simulink model "DrvDem_SelectParameter"  (R2016b)
settings: configuration reference "CodeGenConfigSet" (kept outside this file)
values from neighbouring files (symbols this model uses):
  DrvDem_dnAccLim_CUR = Calibration.Parameter    [init_DrvDem_SelectParameter.m]
  DrvDem_dnAccLim_CURX = Calibration.Parameter    [init_DrvDem_SelectParameter.m]
  DrvDem_dnDeclLim_CUR = Calibration.Parameter    [init_DrvDem_SelectParameter.m]
  DrvDem_dnDeclLim_CURX = Calibration.Parameter    [init_DrvDem_SelectParameter.m]
  DrvDem_facFdbkTrqLosHiParSet_CUR = Calibration.Parameter    [init_DrvDem_SelectParameter.m]
  DrvDem_facFdbkTrqLosHiParSet_CURX = Calibration.Parameter    [init_DrvDem_SelectParameter.m]
  DrvDem_facFdbkTrqLosLoParSet_CUR = Calibration.Parameter    [init_DrvDem_SelectParameter.m]
  DrvDem_facFdbkTrqLosLoParSet_CURX = Calibration.Parameter    [init_DrvDem_SelectParameter.m]
  DrvDem_facNAvrgPT1CorFac_C = Calibration.Parameter    [init_DrvDem_SelectParameter.m]
  DrvDem_facTrqPT1CorFac_C = Calibration.Parameter    [init_DrvDem_SelectParameter.m]
  DrvDem_KiCorTempFac_MAP = Calibration.Parameter    [init_DrvDem_SelectParameter.m]
  DrvDem_KiCorTempFac_MAPX = Calibration.Parameter    [init_DrvDem_SelectParameter.m]
  DrvDem_KiCorTempFac_MAPY = Calibration.Parameter    [init_DrvDem_SelectParameter.m]
  DrvDem_KiCorTrqFac_MAP = Calibration.Parameter    [init_DrvDem_SelectParameter.m]
  DrvDem_KiCorTrqFac_MAPX = Calibration.Parameter    [init_DrvDem_SelectParameter.m]
  DrvDem_KiCorTrqFac_MAPY = Calibration.Parameter    [init_DrvDem_SelectParameter.m]
  DrvDem_KpCorTempFac_MAP = Calibration.Parameter    [init_DrvDem_SelectParameter.m]
  DrvDem_KpCorTempFac_MAPX = Calibration.Parameter    [init_DrvDem_SelectParameter.m]
  DrvDem_KpCorTempFac_MAPY = Calibration.Parameter    [init_DrvDem_SelectParameter.m]
  DrvDem_KpCorTrqFac_MAP = Calibration.Parameter    [init_DrvDem_SelectParameter.m]
  DrvDem_KpCorTrqFac_MAPX = Calibration.Parameter    [init_DrvDem_SelectParameter.m]
  DrvDem_KpCorTrqFac_MAPY = Calibration.Parameter    [init_DrvDem_SelectParameter.m]
  DrvDem_ParSetIKiLo_CUR = Calibration.Parameter    [init_DrvDem_SelectParameter.m]
  DrvDem_ParSetIKiLo_CURX = Calibration.Parameter    [init_DrvDem_SelectParameter.m]
  DrvDem_ParSetIKiNegLo_CUR = Calibration.Parameter    [init_DrvDem_SelectParameter.m]
  DrvDem_ParSetIKiNegLo_CURX = Calibration.Parameter    [init_DrvDem_SelectParameter.m]
  DrvDem_ParSetIKiPosLo_CUR = Calibration.Parameter    [init_DrvDem_SelectParameter.m]
  DrvDem_ParSetIKiPosLo_CURX = Calibration.Parameter    [init_DrvDem_SelectParameter.m]
  DrvDem_ParSetInrtVeh_CUR = Calibration.Parameter    [init_DrvDem_SelectParameter.m]
  DrvDem_ParSetInrtVeh_CURX = Calibration.Parameter    [init_DrvDem_SelectParameter.m]
  DrvDem_ParSetIWinNegHi_C = Calibration.Parameter    [init_DrvDem_SelectParameter.m]
  DrvDem_ParSetIWinNegLo_C = Calibration.Parameter    [init_DrvDem_SelectParameter.m]
  DrvDem_ParSetIWinPosHi_C = Calibration.Parameter    [init_DrvDem_SelectParameter.m]
  DrvDem_ParSetIWinPosLo_C = Calibration.Parameter    [init_DrvDem_SelectParameter.m]
  DrvDem_ParSetPKpLo_CUR = Calibration.Parameter    [init_DrvDem_SelectParameter.m]
  DrvDem_ParSetPKpLo_CURX = Calibration.Parameter    [init_DrvDem_SelectParameter.m]
  DrvDem_ParSetPKpNegLo_CUR = Calibration.Parameter    [init_DrvDem_SelectParameter.m]
  DrvDem_ParSetPKpNegLo_CURX = Calibration.Parameter    [init_DrvDem_SelectParameter.m]
  DrvDem_ParSetPKpPosLo_CUR = Calibration.Parameter    [init_DrvDem_SelectParameter.m]
  DrvDem_ParSetPKpPosLo_CURX = Calibration.Parameter    [init_DrvDem_SelectParameter.m]
  DrvDem_ParSetPWinNegHi_C = Calibration.Parameter    [init_DrvDem_SelectParameter.m]
  DrvDem_ParSetPWinNegLo_C = Calibration.Parameter    [init_DrvDem_SelectParameter.m]
  DrvDem_ParSetPWinPosHi_C = Calibration.Parameter    [init_DrvDem_SelectParameter.m]
  DrvDem_ParSetPWinPosLo_C = Calibration.Parameter    [init_DrvDem_SelectParameter.m]
  DrvDem_ParSetTiFltTrqLos_CUR = Calibration.Parameter    [init_DrvDem_SelectParameter.m]
  DrvDem_ParSetTiFltTrqLos_CURX = Calibration.Parameter    [init_DrvDem_SelectParameter.m]
  DrvDem_swtTempSelParAdap_C = Calibration.Parameter    [init_DrvDem_SelectParameter.m]
  DrvDem_swtTrqSelCorFac_C = Calibration.Parameter    [init_DrvDem_SelectParameter.m]
undefined symbols (not defined in the file or in its folder): DrvDem_SelectParameter_DT, HLSDem_KpCorFac_MAPX
libraries: CXLib x4
settings Model: Creator=lenovo  LastModifiedBy=xuxingpei
settings ConfigSetRef: SourceLocation=Base Workspace

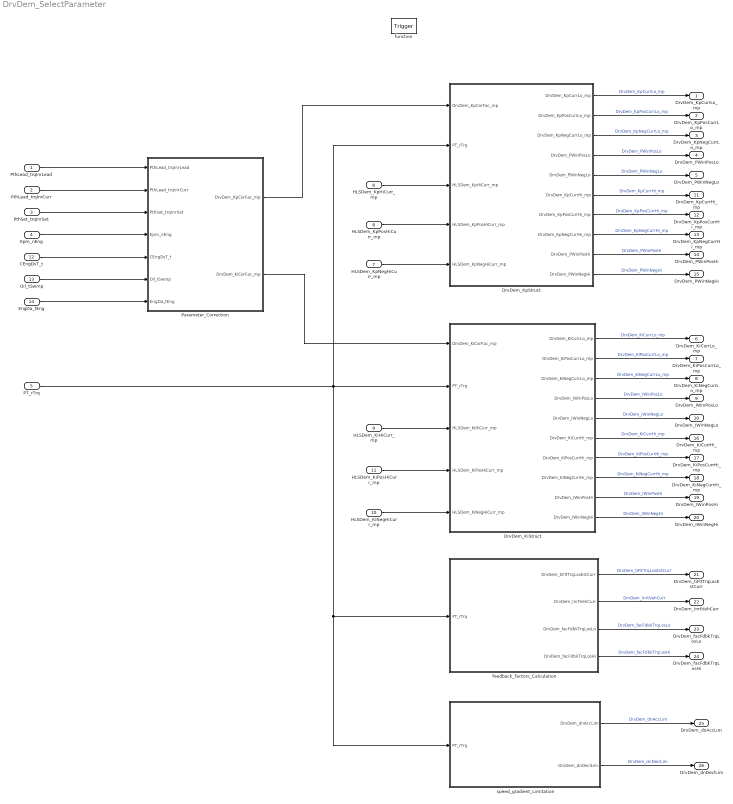
== system DrvDem_SelectParameter ==
  PthLead_trqInrLead : Inport  Tag=Nm  Description=Inner torque lead value  OutMin=-3000  OutMax=3000  OutDataTypeStr=Trq_Nm
  PthLead_trqInrCurr : Inport  Tag=Nm  Description=Actual percent engine torque  Port=2  OutMin=-3000  OutMax=3000  OutDataTypeStr=Trq_Nm
  PthSet_trqInrSet : Inport  Tag=Nm  Description=Inner torque set value after monitoring limitation  Port=3  OutMin=-3000  OutMax=3276.7  OutDataTypeStr=Trq_Nm
  Epm_nEng : Inport  Tag=rpm  Description=Engine speed  Port=4  OutMin=0  OutMax=6000  OutDataTypeStr=EngSpeed_rpm
  PT_rTrq : Inport  Description=Powertrain torque ratio  Port=5  OutMin=-100  OutMax=100  OutDataTypeStr=TransRatio
  HLSDem_KpHiCurr_mp : Inport  Tag=Nm/rpm  Description=Current gain of the P-element of upper path  Port=6  OutMin=-10000  OutMax=10000  OutDataTypeStr=HLSDem_Kp
  HLSDem_KpNegHiCurr_mp : Inport  Tag=Nm/rpm  Description=Current negative large signal gain of the P-element of upper path  Port=7  OutMin=-10000  OutMax=10000  OutDataTypeStr=HLSDem_Kp
  HLSDem_KpPosHiCurr_mp : Inport  Tag=Nm/rpm  Description=Current positive large signal gain of the P-element of upper path  Port=8  OutMin=-10000  OutMax=10000  OutDataTypeStr=HLSDem_Kp
  HLSDem_KiHiCurr_mp : Inport  Tag=Nm/(rpm*s)  Description=Current small signal gain for the I component upper PI - path  Port=9  OutMin=-18000  OutMax=18000  OutDataTypeStr=HLSDem_Ki
  HLSDem_KiNegHiCurr_mp : Inport  Tag=Nm/(rpm*s)  Description=Current negative large signal gain for the I component upper PI - path  Port=10  OutMin=-18000  OutMax=18000  OutDataTypeStr=HLSDem_Ki
  HLSDem_KiPosHiCurr_mp : Inport  Tag=Nm/(rpm*s)  Description=Current positive large signal gain for the I component upper PI-path  Port=11  OutMin=-18000  OutMax=18000  OutDataTypeStr=HLSDem_Ki
  CEngDsT_t : Inport  Tag=deg  Description=engine coolant temperature after filter  Port=12  OutMin=-200  OutMax=200  OutDataTypeStr=Temp_deg
  Oil_tSwmp : Inport  Tag=deg  Description=Oil temperature in oil sump  Port=13  OutMin=-50  OutMax=200  OutDataTypeStr=Temp_deg
  EngDa_tEng : Inport  Tag=deg  Description=Engine temperature  Port=14  OutMin=-1000  OutMax=1000  OutDataTypeStr=Temp_deg
  function : TriggerPort  TriggerType=function-call  VariantControl=Variant
  DrvDem_KiStruct : Subsystem
  DrvDem_KpStruct : Subsystem
  Parameter_Correction : Subsystem
  feedback_factors_Calculation : Subsystem
  speed_gradient_Limitation : Subsystem
  DrvDem_KpCurrLo_mp : Outport  Tag=Nm/rpm  Description=Current gain for the P element for the lower path  OutMin=-10000  OutMax=10000  OutDataTypeStr=HLSDem_Kp
  DrvDem_KpPosCurrLo_mp : Outport  Tag=Nm/rpm  Description=Current positive large signal gain for the P component lower PI-path  Port=2  OutMin=-10000  OutMax=10000  OutDataTypeStr=HLSDem_Kp
  DrvDem_KpNegCurrLo_mp : Outport  Tag=Nm/rpm  Description=Current negative large signal gain for the P component lower PI-path  Port=3  OutMin=-10000  OutMax=10000  OutDataTypeStr=HLSDem_Kp
  DrvDem_PWinPosLo : Outport  Tag=rpm  Description=P component Positive window for parameterset lower PI- path  Port=4  OutMin=-6000  OutMax=6000  OutDataTypeStr=EngSpeed_rpm
  DrvDem_PWinNegLo : Outport  Tag=rpm  Description=P component negative window for parameterset lower PI- path  Port=5  OutMin=-6000  OutMax=6000  OutDataTypeStr=EngSpeed_rpm
  DrvDem_KiCurrLo_mp : Outport  Tag=Nm/(rpm*s)  Description=Current gain for the I element for the lower path  Port=6  OutMin=-18000  OutMax=18000  OutDataTypeStr=HLSDem_Ki
  DrvDem_KiPosCurrLo_mp : Outport  Tag=Nm/(rpm*s)  Description=Current positive large signal gain for the I component lower PI-path  Port=7  OutMin=-18000  OutMax=18000  OutDataTypeStr=HLSDem_Ki
  DrvDem_KiNegCurrLo_mp : Outport  Tag=Nm/(rpm*s)  Description=Current negative large signal gain for the I component lower PI-path  Port=8  OutMin=-18000  OutMax=18000  OutDataTypeStr=HLSDem_Ki
  DrvDem_IWinPosLo : Outport  Tag=rpm  Description=I component Positive window for parameterset lower PI- path  Port=9  OutMin=-6000  OutMax=6000  OutDataTypeStr=EngSpeed_rpm
  DrvDem_IWinNegLo : Outport  Tag=rpm  Description=I component negative window for parameterset lower PI- path  Port=10  OutMin=-6000  OutMax=6000  OutDataTypeStr=EngSpeed_rpm
  DrvDem_KpCurrHi_mp : Outport  Tag=Nm/rpm  Description=Current gain for the P element for the upper path  Port=11  OutMin=-10000  OutMax=10000  OutDataTypeStr=HLSDem_Kp
  DrvDem_KpPosCurrHi_mp : Outport  Tag=Nm/rpm  Description=Current positive large signal gain for the P component upper PI-path  Port=12  OutMin=-10000  OutMax=10000  OutDataTypeStr=HLSDem_Kp
  DrvDem_KpNegCurrHi_mp : Outport  Tag=Nm/rpm  Description=Current negative large signal gain for the P component upper PI-path  Port=13  OutMin=-10000  OutMax=10000  OutDataTypeStr=HLSDem_Kp
  DrvDem_PWinPosHi : Outport  Tag=rpm  Description=P component Positive window for parameterset upper PI- path  Port=14  OutMin=-6000  OutMax=6000  OutDataTypeStr=EngSpeed_rpm
  DrvDem_PWinNegHi : Outport  Tag=rpm  Description=P component negative window for parameterset upper PI- path  Port=15  OutMin=-6000  OutMax=6000  OutDataTypeStr=EngSpeed_rpm
  DrvDem_KiCurrHi_mp : Outport  Tag=Nm/(rpm*s)  Description=Current gain for the I element for the upper path  Port=16  OutMin=-18000  OutMax=18000  OutDataTypeStr=HLSDem_Ki
  DrvDem_KiPosCurrHi_mp : Outport  Tag=Nm/(rpm*s)  Description=Current positive large signal gain for the I component upper PI-path  Port=17  OutMin=-18000  OutMax=18000  OutDataTypeStr=HLSDem_Ki
  DrvDem_KiNegCurrHi_mp : Outport  Tag=Nm/(rpm*s)  Description=Current negative large signal gain for the I component upper PI-path  Port=18  OutMin=-18000  OutMax=18000  OutDataTypeStr=HLSDem_Ki
  DrvDem_IWinPosHi : Outport  Tag=rpm  Description=I component Positive window for parameterset upper PI- path  Port=19  OutMin=-6000  OutMax=6000  OutDataTypeStr=EngSpeed_rpm
  DrvDem_IWinNegHi : Outport  Tag=rpm  Description=I component negative window for parameterset upper PI- path  Port=20  OutMin=-6000  OutMax=6000  OutDataTypeStr=EngSpeed_rpm
  DrvDem_tiFltTrqLosEstCurr : Outport  Description=Time constant (PT1filter) for EISGov torque loss estimation  Port=21  OutMin=0  OutMax=99.998  OutDataTypeStr=PT_fac
  DrvDem_InrtVehCurr : Outport  Tag=Nm/(rpm/s)  Description=Mass Inertia for EISGov torque loss estimation  Port=22  OutMin=-50  OutMax=50  OutDataTypeStr=HLSDem_Inrt
  DrvDem_facFdbkTrqLosLo : Outport  Tag=rpm/Nm  Description=Inner feedback factor for the lower setpoint  Port=23  OutMin=-20  OutMax=20  OutDataTypeStr=FdbkNm2rpm_rpm_Nm
  DrvDem_facFdbkTrqLosHi : Outport  Tag=rpm/Nm  Description=Inner feedback factor for the upper setpoint  Port=24  OutMin=-20  OutMax=20  OutDataTypeStr=FdbkNm2rpm_rpm_Nm
  DrvDem_dnAccLim : Outport  Tag=rpm/s  Description=Maximum permissible acceleration (Engine speed)  Port=25  OutMin=-12000  OutMax=12000  OutDataTypeStr=EngSpeed_rpm_s
  DrvDem_dnDeclLim : Outport  Tag=rpm/s  Description=Maximum permissible deceleration (Engine speed)  Port=26  OutMin=-12000  OutMax=12000  OutDataTypeStr=EngSpeed_rpm_s
  wires:
  PthLead_trqInrLead/1 -> Parameter_Correction/1(PthLead_trqInrLead)
  PthLead_trqInrCurr/1 -> Parameter_Correction/2(PthLead_trqInrCurr)
  PthSet_trqInrSet/1 -> Parameter_Correction/3(PthSet_trqInrSet)
  Epm_nEng/1 -> Parameter_Correction/4(Epm_nEng)
  CEngDsT_t/1 -> Parameter_Correction/5(CEngDsT_t)
  Oil_tSwmp/1 -> Parameter_Correction/6(Oil_tSwmp)
  EngDa_tEng/1 -> Parameter_Correction/7(EngDa_tEng)
  PT_rTrq/1 -> speed_gradient_Limitation/1(PT_rTrq), feedback_factors_Calculation/1(PT_rTrq), DrvDem_KpStruct/2(PT_rTrq), DrvDem_KiStruct/2(PT_rTrq)
  Parameter_Correction/1(DrvDem_KpCorFac_mp) -> DrvDem_KpStruct/1(DrvDem_KpCorFac_mp)
  HLSDem_KpHiCurr_mp/1 -> DrvDem_KpStruct/3(HLSDem_KpHiCurr_mp)
  HLSDem_KpPosHiCurr_mp/1 -> DrvDem_KpStruct/4(HLSDem_KpPosHiCurr_mp)
  HLSDem_KpNegHiCurr_mp/1 -> DrvDem_KpStruct/5(HLSDem_KpNegHiCurr_mp)
  DrvDem_KpStruct/1(DrvDem_KpCurrLo_mp) -> DrvDem_KpCurrLo_mp/1  "DrvDem_KpCurrLo_mp"
  DrvDem_KpStruct/2(DrvDem_KpPosCurrLo_mp) -> DrvDem_KpPosCurrLo_mp/1  "DrvDem_KpPosCurrLo_mp"
  DrvDem_KpStruct/3(DrvDem_KpNegCurrLo_mp) -> DrvDem_KpNegCurrLo_mp/1  "DrvDem_KpNegCurrLo_mp"
  DrvDem_KpStruct/4(DrvDem_PWinPosLo) -> DrvDem_PWinPosLo/1  "DrvDem_PWinPosLo"
  DrvDem_KpStruct/5(DrvDem_PWinNegLo) -> DrvDem_PWinNegLo/1  "DrvDem_PWinNegLo"
  DrvDem_KpStruct/6(DrvDem_KpCurrHi_mp) -> DrvDem_KpCurrHi_mp/1  "DrvDem_KpCurrHi_mp"
  DrvDem_KpStruct/7(DrvDem_KpPosCurrHi_mp) -> DrvDem_KpPosCurrHi_mp/1  "DrvDem_KpPosCurrHi_mp"
  DrvDem_KpStruct/8(DrvDem_KpNegCurrHi_mp) -> DrvDem_KpNegCurrHi_mp/1  "DrvDem_KpNegCurrHi_mp"
  DrvDem_KpStruct/9(DrvDem_PWinPosHi) -> DrvDem_PWinPosHi/1  "DrvDem_PWinPosHi"
  DrvDem_KpStruct/10(DrvDem_PWinNegHi) -> DrvDem_PWinNegHi/1  "DrvDem_PWinNegHi"
  HLSDem_KiHiCurr_mp/1 -> DrvDem_KiStruct/3(HLSDem_KiHiCurr_mp)
  DrvDem_KiStruct/1(DrvDem_KiCurrLo_mp) -> DrvDem_KiCurrLo_mp/1  "DrvDem_KiCurrLo_mp"
  DrvDem_KiStruct/2(DrvDem_KiPosCurrLo_mp) -> DrvDem_KiPosCurrLo_mp/1  "DrvDem_KiPosCurrLo_mp"
  DrvDem_KiStruct/3(DrvDem_KiNegCurrLo_mp) -> DrvDem_KiNegCurrLo_mp/1  "DrvDem_KiNegCurrLo_mp"
  DrvDem_KiStruct/4(DrvDem_IWinPosLo) -> DrvDem_IWinPosLo/1  "DrvDem_IWinPosLo"
  DrvDem_KiStruct/5(DrvDem_IWinNegLo) -> DrvDem_IWinNegLo/1  "DrvDem_IWinNegLo"
  DrvDem_KiStruct/6(DrvDem_KiCurrHi_mp) -> DrvDem_KiCurrHi_mp/1  "DrvDem_KiCurrHi_mp"
  DrvDem_KiStruct/7(DrvDem_KiPosCurrHi_mp) -> DrvDem_KiPosCurrHi_mp/1  "DrvDem_KiPosCurrHi_mp"
  DrvDem_KiStruct/8(DrvDem_KiNegCurrHi_mp) -> DrvDem_KiNegCurrHi_mp/1  "DrvDem_KiNegCurrHi_mp"
  DrvDem_KiStruct/9(DrvDem_IWinPosHi) -> DrvDem_IWinPosHi/1  "DrvDem_IWinPosHi"
  DrvDem_KiStruct/10(DrvDem_IWinNegHi) -> DrvDem_IWinNegHi/1  "DrvDem_IWinNegHi"
  feedback_factors_Calculation/1(DrvDem_tiFltTrqLosEstCurr) -> DrvDem_tiFltTrqLosEstCurr/1  "DrvDem_tiFltTrqLosEstCurr"
  feedback_factors_Calculation/2(DrvDem_InrtVehCurr) -> DrvDem_InrtVehCurr/1  "DrvDem_InrtVehCurr"
  feedback_factors_Calculation/3(DrvDem_facFdbkTrqLosLo) -> DrvDem_facFdbkTrqLosLo/1  "DrvDem_facFdbkTrqLosLo"
  feedback_factors_Calculation/4(DrvDem_facFdbkTrqLosHi) -> DrvDem_facFdbkTrqLosHi/1  "DrvDem_facFdbkTrqLosHi"
  speed_gradient_Limitation/1(DrvDem_dnAccLim) -> DrvDem_dnAccLim/1  "DrvDem_dnAccLim"
  speed_gradient_Limitation/2(DrvDem_dnDeclLim) -> DrvDem_dnDeclLim/1  "DrvDem_dnDeclLim"
  Parameter_Correction/2(DrvDem_KiCorFac_mp) -> DrvDem_KiStruct/1(DrvDem_KiCorFac_mp)
  HLSDem_KiPosHiCurr_mp/1 -> DrvDem_KiStruct/4(HLSDem_KiPosHiCurr_mp)
  HLSDem_KiNegHiCurr_mp/1 -> DrvDem_KiStruct/5(HLSDem_KiNegHiCurr_mp)

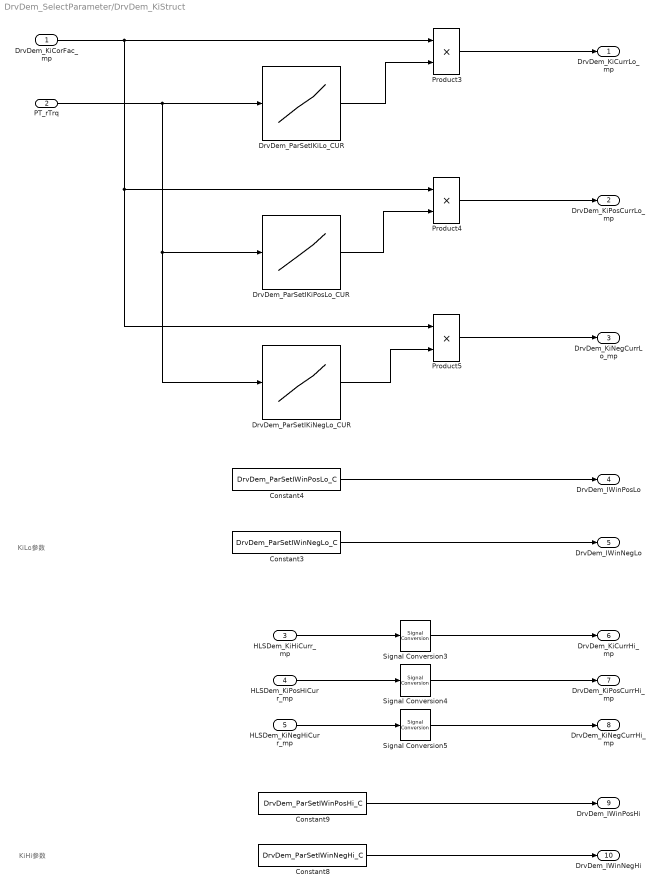
== system DrvDem_SelectParameter/DrvDem_KiStruct ==
  note: KiLo参数
  note: KiHi参数
  DrvDem_KiCorFac_mp : Inport
  PT_rTrq : Inport  Port=2
  HLSDem_KiHiCurr_mp : Inport  Tag=Nm/(rpm*s)  Description=Current small signal gain for the I component upper PI - path  Port=3
  HLSDem_KiPosHiCurr_mp : Inport  Tag=Nm/(rpm*s)  Description=Current positive large signal gain for the I component upper PI-path  Port=4
  HLSDem_KiNegHiCurr_mp : Inport  Tag=Nm/(rpm*s)  Description=Current negative large signal gain for the I component upper PI - path  Port=5
  Constant3 : Constant  Value=DrvDem_ParSetIWinNegLo_C  SampleTime=-1
  Constant4 : Constant  Value=DrvDem_ParSetIWinPosLo_C  SampleTime=-1
  Constant8 : Constant  Value=DrvDem_ParSetIWinNegHi_C  SampleTime=-1
  Constant9 : Constant  Value=DrvDem_ParSetIWinPosHi_C  SampleTime=-1
  DrvDem_ParSetIKiLo_CUR : Lookup_n-D  NumberOfTableDimensions=1  BreakpointsForDimension1=DrvDem_ParSetIKiLo_CURX  BreakpointsForDimension2=HLSDem_KpCorFac_MAPX  Table=DrvDem_ParSetIKiLo_CUR  ExtrapMethod=Clip  InternalRulePriority=Speed  OutDataTypeStr=Inherit: Inherit via back propagation  RndMeth=Simplest  SaturateOnIntegerOverflow=on
  DrvDem_ParSetIKiNegLo_CUR : Lookup_n-D  NumberOfTableDimensions=1  BreakpointsForDimension1=DrvDem_ParSetIKiNegLo_CURX  BreakpointsForDimension2=HLSDem_KpCorFac_MAPX  Table=DrvDem_ParSetIKiNegLo_CUR  ExtrapMethod=Clip  InternalRulePriority=Speed  OutDataTypeStr=Inherit: Inherit via back propagation  RndMeth=Simplest  SaturateOnIntegerOverflow=on
  DrvDem_ParSetIKiPosLo_CUR : Lookup_n-D  NumberOfTableDimensions=1  BreakpointsForDimension1=DrvDem_ParSetIKiPosLo_CURX  BreakpointsForDimension2=HLSDem_KpCorFac_MAPX  Table=DrvDem_ParSetIKiPosLo_CUR  ExtrapMethod=Clip  InternalRulePriority=Speed  OutDataTypeStr=Inherit: Inherit via back propagation  RndMeth=Simplest  SaturateOnIntegerOverflow=on
  Product3 : Product  OutDataTypeStr=Inherit: Inherit via back propagation
  Product4 : Product  OutDataTypeStr=Inherit: Inherit via back propagation
  Product5 : Product  OutDataTypeStr=Inherit: Inherit via back propagation
  Signal Conversion3 : SignalConversion  OverrideOpt=off
  Signal Conversion4 : SignalConversion  OverrideOpt=off
  Signal Conversion5 : SignalConversion  OverrideOpt=off
  DrvDem_KiCurrLo_mp : Outport  Tag=Nm/(rpm*s)  Description=Current gain for the I element for the lower path  OutMin=-18000  OutMax=18000  OutDataTypeStr=HLSDem_Ki
  DrvDem_KiPosCurrLo_mp : Outport  Tag=Nm/(rpm*s)  Description=Current positive large signal gain for the I component lower PI-path  Port=2  OutMin=-18000  OutMax=18000  OutDataTypeStr=HLSDem_Ki
  DrvDem_KiNegCurrLo_mp : Outport  Tag=Nm/(rpm*s)  Description=Current negative large signal gain for the I component lower PI-path  Port=3  OutMin=-18000  OutMax=18000  OutDataTypeStr=HLSDem_Ki
  DrvDem_IWinPosLo : Outport  Tag=rpm  Description=I component Positive window for parameterset lower PI- path  Port=4  OutMin=-6000  OutMax=6000  OutDataTypeStr=EngSpeed_rpm
  DrvDem_IWinNegLo : Outport  Tag=rpm  Description=I component negative window for parameterset lower PI- path  Port=5  OutMin=-6000  OutMax=6000  OutDataTypeStr=EngSpeed_rpm
  DrvDem_KiCurrHi_mp : Outport  Tag=Nm/(rpm*s)  Description=Current gain for the I element for the upper path  Port=6  OutMin=-18000  OutMax=18000  OutDataTypeStr=HLSDem_Ki
  DrvDem_KiPosCurrHi_mp : Outport  Tag=Nm/(rpm*s)  Description=Current positive large signal gain for the I component upper PI-path  Port=7  OutMin=-18000  OutMax=18000  OutDataTypeStr=HLSDem_Ki
  DrvDem_KiNegCurrHi_mp : Outport  Tag=Nm/(rpm*s)  Description=Current negative large signal gain for the I component upper PI-path  Port=8  OutMin=-18000  OutMax=18000  OutDataTypeStr=HLSDem_Ki
  DrvDem_IWinPosHi : Outport  Tag=rpm  Description=I component Positive window for parameterset upper PI- path  Port=9  OutMin=-6000  OutMax=6000  OutDataTypeStr=EngSpeed_rpm
  DrvDem_IWinNegHi : Outport  Tag=rpm  Description=I component negative window for parameterset upper PI- path  Port=10  OutMin=-6000  OutMax=6000  OutDataTypeStr=EngSpeed_rpm
  wires:
  PT_rTrq/1 -> DrvDem_ParSetIKiNegLo_CUR/1, DrvDem_ParSetIKiPosLo_CUR/1, DrvDem_ParSetIKiLo_CUR/1
  Product3/1 -> DrvDem_KiCurrLo_mp/1
  Product4/1 -> DrvDem_KiPosCurrLo_mp/1
  Product5/1 -> DrvDem_KiNegCurrLo_mp/1
  Constant4/1 -> DrvDem_IWinPosLo/1
  Constant3/1 -> DrvDem_IWinNegLo/1
  Signal Conversion3/1 -> DrvDem_KiCurrHi_mp/1
  Signal Conversion4/1 -> DrvDem_KiPosCurrHi_mp/1
  Signal Conversion5/1 -> DrvDem_KiNegCurrHi_mp/1
  DrvDem_ParSetIKiNegLo_CUR/1 -> Product5/2
  DrvDem_KiCorFac_mp/1 -> Product5/1, Product4/1, Product3/1
  DrvDem_ParSetIKiLo_CUR/1 -> Product3/2
  DrvDem_ParSetIKiPosLo_CUR/1 -> Product4/2
  HLSDem_KiHiCurr_mp/1 -> Signal Conversion3/1
  Constant8/1 -> DrvDem_IWinNegHi/1
  Constant9/1 -> DrvDem_IWinPosHi/1
  HLSDem_KiNegHiCurr_mp/1 -> Signal Conversion5/1
  HLSDem_KiPosHiCurr_mp/1 -> Signal Conversion4/1

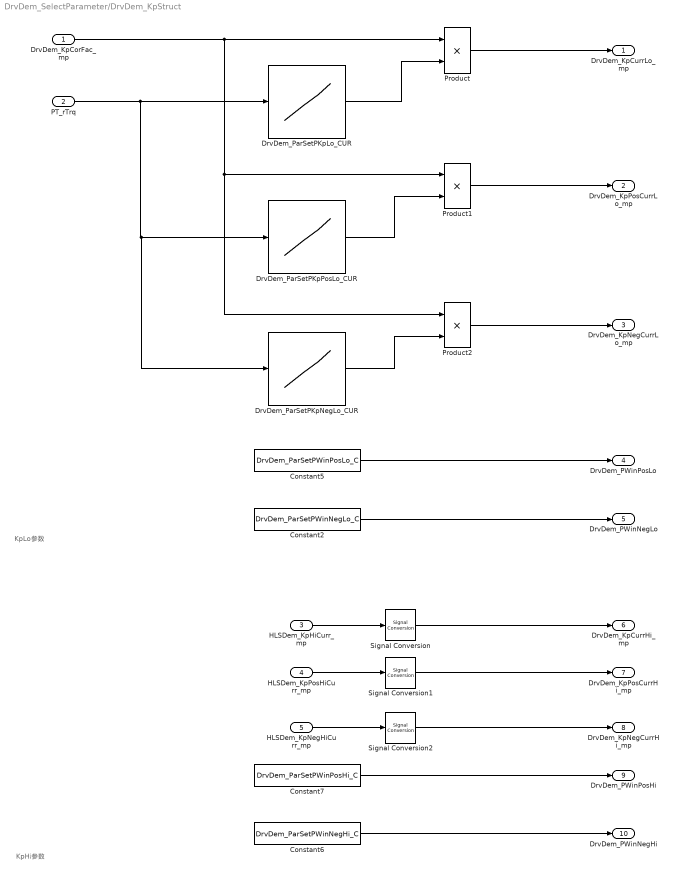
== system DrvDem_SelectParameter/DrvDem_KpStruct ==
  note: KpLo参数
  note: KpHi参数
  DrvDem_KpCorFac_mp : Inport
  PT_rTrq : Inport  Port=2
  HLSDem_KpHiCurr_mp : Inport  Tag=Nm/rpm  Description=Current gain of the P-element of upper path  Port=3
  HLSDem_KpPosHiCurr_mp : Inport  Tag=Nm/rpm  Description=Current positive large signal gain of the P-element of upper path  Port=4
  HLSDem_KpNegHiCurr_mp : Inport  Tag=Nm/rpm  Description=Current negative large signal gain of the P-element of upper path  Port=5
  Constant2 : Constant  Value=DrvDem_ParSetPWinNegLo_C  SampleTime=-1
  Constant5 : Constant  Value=DrvDem_ParSetPWinPosLo_C  SampleTime=-1
  Constant6 : Constant  Value=DrvDem_ParSetPWinNegHi_C  SampleTime=-1
  Constant7 : Constant  Value=DrvDem_ParSetPWinPosHi_C  SampleTime=-1
  DrvDem_ParSetPKpLo_CUR : Lookup_n-D  NumberOfTableDimensions=1  BreakpointsForDimension1=DrvDem_ParSetPKpLo_CURX  BreakpointsForDimension2=HLSDem_KpCorFac_MAPX  Table=DrvDem_ParSetPKpLo_CUR  ExtrapMethod=Clip  InternalRulePriority=Speed  OutDataTypeStr=Inherit: Inherit via back propagation  RndMeth=Simplest  SaturateOnIntegerOverflow=on
  DrvDem_ParSetPKpNegLo_CUR : Lookup_n-D  NumberOfTableDimensions=1  BreakpointsForDimension1=DrvDem_ParSetPKpNegLo_CURX  BreakpointsForDimension2=HLSDem_KpCorFac_MAPX  Table=DrvDem_ParSetPKpNegLo_CUR  ExtrapMethod=Clip  InternalRulePriority=Speed  OutDataTypeStr=Inherit: Inherit via back propagation  RndMeth=Simplest  SaturateOnIntegerOverflow=on
  DrvDem_ParSetPKpPosLo_CUR : Lookup_n-D  NumberOfTableDimensions=1  BreakpointsForDimension1=DrvDem_ParSetPKpPosLo_CURX  BreakpointsForDimension2=HLSDem_KpCorFac_MAPX  Table=DrvDem_ParSetPKpPosLo_CUR  ExtrapMethod=Clip  InternalRulePriority=Speed  OutDataTypeStr=Inherit: Inherit via back propagation  RndMeth=Simplest  SaturateOnIntegerOverflow=on
  Product : Product  OutDataTypeStr=Inherit: Inherit via back propagation
  Product1 : Product  OutDataTypeStr=Inherit: Inherit via back propagation
  Product2 : Product  OutDataTypeStr=Inherit: Inherit via back propagation
  Signal Conversion : SignalConversion  OverrideOpt=off
  Signal Conversion1 : SignalConversion  OverrideOpt=off
  Signal Conversion2 : SignalConversion  OverrideOpt=off
  DrvDem_KpCurrLo_mp : Outport  Tag=Nm/rpm  Description=Current gain for the P element for the lower path  OutMin=-10000  OutMax=10000  OutDataTypeStr=HLSDem_Kp
  DrvDem_KpPosCurrLo_mp : Outport  Tag=Nm/rpm  Description=Current positive large signal gain for the P component lower PI-path  Port=2  OutMin=-10000  OutMax=10000  OutDataTypeStr=HLSDem_Kp
  DrvDem_KpNegCurrLo_mp : Outport  Tag=Nm/rpm  Description=Current negative large signal gain for the P component lower PI-path  Port=3  OutMin=-10000  OutMax=10000  OutDataTypeStr=HLSDem_Kp
  DrvDem_PWinPosLo : Outport  Tag=rpm  Description=P component Positive window for parameterset lower PI- path  Port=4  OutMin=-6000  OutMax=6000  OutDataTypeStr=EngSpeed_rpm
  DrvDem_PWinNegLo : Outport  Tag=rpm  Description=P component negative window for parameterset lower PI- path  Port=5  OutMin=-6000  OutMax=6000  OutDataTypeStr=EngSpeed_rpm
  DrvDem_KpCurrHi_mp : Outport  Tag=Nm/rpm  Description=Current gain for the P element for the upper path  Port=6  OutMin=-10000  OutMax=10000  OutDataTypeStr=HLSDem_Kp
  DrvDem_KpPosCurrHi_mp : Outport  Tag=Nm/rpm  Description=Current positive large signal gain for the P component upper PI-path  Port=7  OutMin=-10000  OutMax=10000  OutDataTypeStr=HLSDem_Kp
  DrvDem_KpNegCurrHi_mp : Outport  Tag=Nm/rpm  Description=Current negative large signal gain for the P component upper PI-path  Port=8  OutMin=-10000  OutMax=10000  OutDataTypeStr=HLSDem_Kp
  DrvDem_PWinPosHi : Outport  Tag=rpm  Description=P component Positive window for parameterset upper PI- path  Port=9  OutMin=-6000  OutMax=6000  OutDataTypeStr=EngSpeed_rpm
  DrvDem_PWinNegHi : Outport  Tag=rpm  Description=P component negative window for parameterset upper PI- path  Port=10  OutMin=-6000  OutMax=6000  OutDataTypeStr=EngSpeed_rpm
  wires:
  Product/1 -> DrvDem_KpCurrLo_mp/1
  Product1/1 -> DrvDem_KpPosCurrLo_mp/1
  Product2/1 -> DrvDem_KpNegCurrLo_mp/1
  Signal Conversion/1 -> DrvDem_KpCurrHi_mp/1
  Signal Conversion1/1 -> DrvDem_KpPosCurrHi_mp/1
  Signal Conversion2/1 -> DrvDem_KpNegCurrHi_mp/1
  Constant7/1 -> DrvDem_PWinPosHi/1
  Constant6/1 -> DrvDem_PWinNegHi/1
  DrvDem_ParSetPKpNegLo_CUR/1 -> Product2/2
  DrvDem_ParSetPKpLo_CUR/1 -> Product/2
  HLSDem_KpHiCurr_mp/1 -> Signal Conversion/1
  HLSDem_KpPosHiCurr_mp/1 -> Signal Conversion1/1
  DrvDem_ParSetPKpPosLo_CUR/1 -> Product1/2
  HLSDem_KpNegHiCurr_mp/1 -> Signal Conversion2/1
  DrvDem_KpCorFac_mp/1 -> Product/1, Product2/1, Product1/1
  PT_rTrq/1 -> DrvDem_ParSetPKpNegLo_CUR/1, DrvDem_ParSetPKpPosLo_CUR/1, DrvDem_ParSetPKpLo_CUR/1
  Constant5/1 -> DrvDem_PWinPosLo/1
  Constant2/1 -> DrvDem_PWinNegLo/1

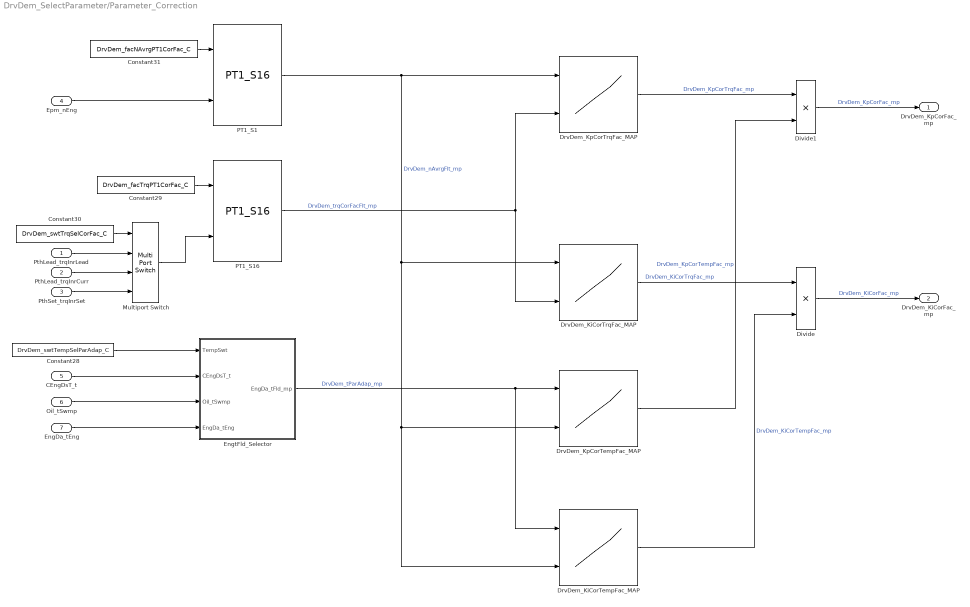
== system DrvDem_SelectParameter/Parameter_Correction ==
  PthLead_trqInrLead : Inport  Tag=Nm  Description=Inner torque lead value  OutMin=-3000  OutMax=3000  OutDataTypeStr=Trq_Nm
  PthLead_trqInrCurr : Inport  Tag=Nm  Description=Actual percent engine torque  Port=2  OutMin=-3000  OutMax=3000  OutDataTypeStr=Trq_Nm
  PthSet_trqInrSet : Inport  Tag=Nm  Description=Inner torque set value after monitoring limitation  Port=3  OutMin=-3000  OutMax=3276.7  OutDataTypeStr=Trq_Nm
  Epm_nEng : Inport  Tag=rpm  Description=Engine speed  Port=4  OutMin=0  OutMax=6000  OutDataTypeStr=EngSpeed_rpm
  CEngDsT_t : Inport  Tag=deg  Description=engine coolant temperature after filter  Port=5  OutMin=-200  OutMax=200  OutDataTypeStr=Temp_deg
  Oil_tSwmp : Inport  Tag=deg  Description=Oil temperature in oil sump  Port=6  OutMin=-50  OutMax=200  OutDataTypeStr=Temp_deg
  EngDa_tEng : Inport  Tag=deg  Description=Engine temperature  Port=7  OutMin=-1000  OutMax=1000  OutDataTypeStr=Temp_deg
  Constant28 : Constant  Value=DrvDem_swtTempSelParAdap_C
  Constant29 : Constant  Value=DrvDem_facTrqPT1CorFac_C
  Constant30 : Constant  Value=DrvDem_swtTrqSelCorFac_C
  Constant31 : Constant  Value=DrvDem_facNAvrgPT1CorFac_C
  Divide : Product  Inputs=**  OutDataTypeStr=Inherit: Inherit via back propagation  SaturateOnIntegerOverflow=on
  Divide1 : Product  Inputs=**  OutDataTypeStr=Inherit: Inherit via back propagation  SaturateOnIntegerOverflow=on
  DrvDem_KiCorTempFac_MAP : Lookup_n-D  RequirementInfo={} %GIDa_4a937b4a_64a0_4536_bc1d_590dfe089b74  DialogController=Simulink.DDGSource  BreakpointsForDimension1=DrvDem_KiCorTempFac_MAPY  BreakpointsForDimension2=DrvDem_KiCorTempFac_MAPX  IndexSearchMethod=Linear search  BeginIndexSearchUsingPreviousIndexResult=on  Table=DrvDem_KiCorTempFac_MAP  ExtrapMethod=Clip  UseLastTableValue=on  InternalRulePriority=Speed  OutDataTypeStr=Inherit: Inherit via back propagation  SaturateOnIntegerOverflow=on
  DrvDem_KiCorTrqFac_MAP : Lookup_n-D  RequirementInfo={} %GIDa_f38336a6_d113_464b_a9ad_fd3b7786cf7d  DialogController=Simulink.DDGSource  BreakpointsForDimension1=DrvDem_KiCorTrqFac_MAPY  BreakpointsForDimension2=DrvDem_KiCorTrqFac_MAPX  IndexSearchMethod=Linear search  BeginIndexSearchUsingPreviousIndexResult=on  Table=DrvDem_KiCorTrqFac_MAP  ExtrapMethod=Clip  UseLastTableValue=on  InternalRulePriority=Speed  OutDataTypeStr=Inherit: Inherit via back propagation  SaturateOnIntegerOverflow=on
  DrvDem_KpCorTempFac_MAP : Lookup_n-D  RequirementInfo={} %GIDa_f110a671_925f_41cd_a2c0_5fdf25a792e7  DialogController=Simulink.DDGSource  BreakpointsForDimension1=DrvDem_KpCorTempFac_MAPY  BreakpointsForDimension2=DrvDem_KpCorTempFac_MAPX  IndexSearchMethod=Linear search  BeginIndexSearchUsingPreviousIndexResult=on  Table=DrvDem_KpCorTempFac_MAP  ExtrapMethod=Clip  UseLastTableValue=on  InternalRulePriority=Speed  OutDataTypeStr=Inherit: Inherit via back propagation  SaturateOnIntegerOverflow=on
  DrvDem_KpCorTrqFac_MAP : Lookup_n-D  RequirementInfo={} %GIDa_b3bf7277_cb88_4303_8557_7656cedc9791  DialogController=Simulink.DDGSource  BreakpointsForDimension1=DrvDem_KpCorTrqFac_MAPY  BreakpointsForDimension2=DrvDem_KpCorTrqFac_MAPX  IndexSearchMethod=Linear search  BeginIndexSearchUsingPreviousIndexResult=on  Table=DrvDem_KpCorTrqFac_MAP  ExtrapMethod=Clip  UseLastTableValue=on  InternalRulePriority=Speed  OutDataTypeStr=Inherit: Inherit via back propagation  SaturateOnIntegerOverflow=on
  EngtFld_Selector : Subsystem
  Multiport Switch : MultiPortSwitch  DataPortOrder=Specify indices  DataPortIndices={2,1,0}  SaturateOnIntegerOverflow=on  InputSameDT=on
  PT1_S1 : CXLib/PT1_S16
  PT1_S16 : CXLib/PT1_S16
  DrvDem_KpCorFac_mp : Outport
  DrvDem_KiCorFac_mp : Outport  Port=2
  wires:
  Constant30/1 -> Multiport Switch/1
  DrvDem_KiCorTrqFac_MAP/1 -> Divide/1  "DrvDem_KiCorTrqFac_mp"
  Constant31/1 -> PT1_S1/1
  DrvDem_KiCorTempFac_MAP/1 -> Divide/2  "DrvDem_KiCorTempFac_mp"
  Constant29/1 -> PT1_S16/1
  PT1_S1/1 -> DrvDem_KiCorTrqFac_MAP/1, DrvDem_KiCorTempFac_MAP/2, DrvDem_KpCorTempFac_MAP/2, DrvDem_KpCorTrqFac_MAP/1  "DrvDem_nAvrgFlt_mp"
  Multiport Switch/1 -> PT1_S16/2
  PthSet_trqInrSet/1 -> Multiport Switch/4
  DrvDem_KpCorTempFac_MAP/1 -> Divide1/2  "DrvDem_KpCorTempFac_mp"
  PT1_S16/1 -> DrvDem_KpCorTrqFac_MAP/2, DrvDem_KiCorTrqFac_MAP/2  "DrvDem_trqCorFacFlt_mp"
  PthLead_trqInrLead/1 -> Multiport Switch/2
  Epm_nEng/1 -> PT1_S1/2
  DrvDem_KpCorTrqFac_MAP/1 -> Divide1/1  "DrvDem_KpCorTrqFac_mp"
  PthLead_trqInrCurr/1 -> Multiport Switch/3
  Divide1/1 -> DrvDem_KpCorFac_mp/1  "DrvDem_KpCorFac_mp"
  Divide/1 -> DrvDem_KiCorFac_mp/1  "DrvDem_KiCorFac_mp"
  Oil_tSwmp/1 -> EngtFld_Selector/3(Oil_tSwmp)
  Constant28/1 -> EngtFld_Selector/1(TempSwt)
  EngtFld_Selector/1(EngDa_tFld_mp) -> DrvDem_KpCorTempFac_MAP/1, DrvDem_KiCorTempFac_MAP/1  "DrvDem_tParAdap_mp"
  EngDa_tEng/1 -> EngtFld_Selector/4(EngDa_tEng)
  CEngDsT_t/1 -> EngtFld_Selector/2(CEngDsT_t)

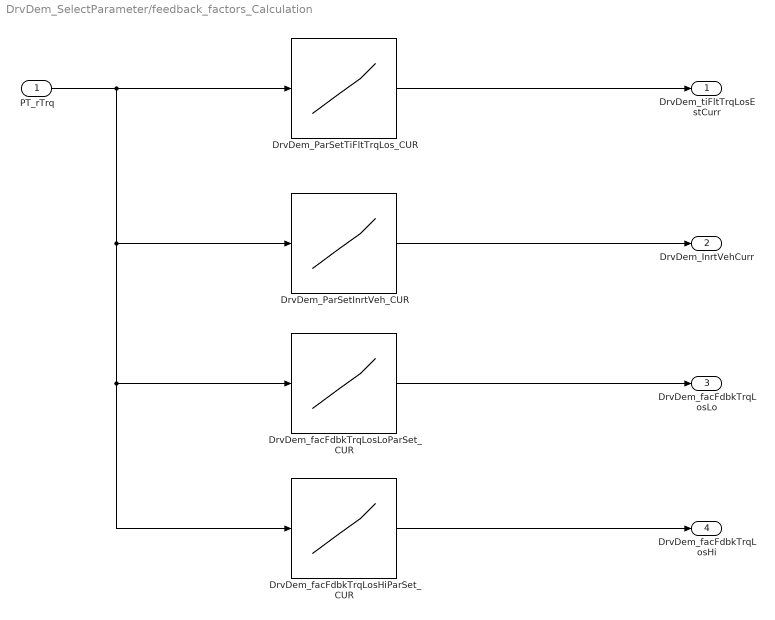
== system DrvDem_SelectParameter/feedback_factors_Calculation ==
  PT_rTrq : Inport
  DrvDem_ParSetInrtVeh_CUR : Lookup_n-D  NumberOfTableDimensions=1  BreakpointsForDimension1=DrvDem_ParSetInrtVeh_CURX  BreakpointsForDimension2=HLSDem_KpCorFac_MAPX  Table=DrvDem_ParSetInrtVeh_CUR  ExtrapMethod=Clip  InternalRulePriority=Speed  OutDataTypeStr=Inherit: Inherit via back propagation  RndMeth=Simplest  SaturateOnIntegerOverflow=on
  DrvDem_ParSetTiFltTrqLos_CUR : Lookup_n-D  NumberOfTableDimensions=1  BreakpointsForDimension1=DrvDem_ParSetTiFltTrqLos_CURX  BreakpointsForDimension2=HLSDem_KpCorFac_MAPX  Table=DrvDem_ParSetTiFltTrqLos_CUR  ExtrapMethod=Clip  InternalRulePriority=Speed  OutDataTypeStr=Inherit: Inherit via back propagation  RndMeth=Simplest  SaturateOnIntegerOverflow=on
  DrvDem_facFdbkTrqLosHiParSet_CUR : Lookup_n-D  NumberOfTableDimensions=1  BreakpointsForDimension1=DrvDem_facFdbkTrqLosHiParSet_CURX  BreakpointsForDimension2=HLSDem_KpCorFac_MAPX  Table=DrvDem_facFdbkTrqLosHiParSet_CUR  ExtrapMethod=Clip  InternalRulePriority=Speed  OutDataTypeStr=Inherit: Inherit via back propagation  RndMeth=Simplest  SaturateOnIntegerOverflow=on
  DrvDem_facFdbkTrqLosLoParSet_CUR : Lookup_n-D  NumberOfTableDimensions=1  BreakpointsForDimension1=DrvDem_facFdbkTrqLosLoParSet_CURX  BreakpointsForDimension2=HLSDem_KpCorFac_MAPX  Table=DrvDem_facFdbkTrqLosLoParSet_CUR  ExtrapMethod=Clip  InternalRulePriority=Speed  OutDataTypeStr=Inherit: Inherit via back propagation  RndMeth=Simplest  SaturateOnIntegerOverflow=on
  DrvDem_tiFltTrqLosEstCurr : Outport  Description=Time constant (PT1filter) for EISGov torque loss estimation  OutMin=0  OutMax=99.998  OutDataTypeStr=PT_fac
  DrvDem_InrtVehCurr : Outport  Tag=Nm/(rpm/s)  Description=Mass Inertia for EISGov torque loss estimation  Port=2  OutMin=-50  OutMax=50  OutDataTypeStr=HLSDem_Inrt
  DrvDem_facFdbkTrqLosLo : Outport  Tag=rpm/Nm  Description=Inner feedback factor for the lower setpoint  Port=3  OutMin=-20  OutMax=20  OutDataTypeStr=FdbkNm2rpm_rpm_Nm
  DrvDem_facFdbkTrqLosHi : Outport  Tag=rpm/Nm  Description=Inner feedback factor for the upper setpoint  Port=4  OutMin=-20  OutMax=20  OutDataTypeStr=FdbkNm2rpm_rpm_Nm
  wires:
  DrvDem_ParSetTiFltTrqLos_CUR/1 -> DrvDem_tiFltTrqLosEstCurr/1
  DrvDem_ParSetInrtVeh_CUR/1 -> DrvDem_InrtVehCurr/1
  DrvDem_facFdbkTrqLosLoParSet_CUR/1 -> DrvDem_facFdbkTrqLosLo/1
  DrvDem_facFdbkTrqLosHiParSet_CUR/1 -> DrvDem_facFdbkTrqLosHi/1
  PT_rTrq/1 -> DrvDem_facFdbkTrqLosHiParSet_CUR/1, DrvDem_facFdbkTrqLosLoParSet_CUR/1, DrvDem_ParSetInrtVeh_CUR/1, DrvDem_ParSetTiFltTrqLos_CUR/1

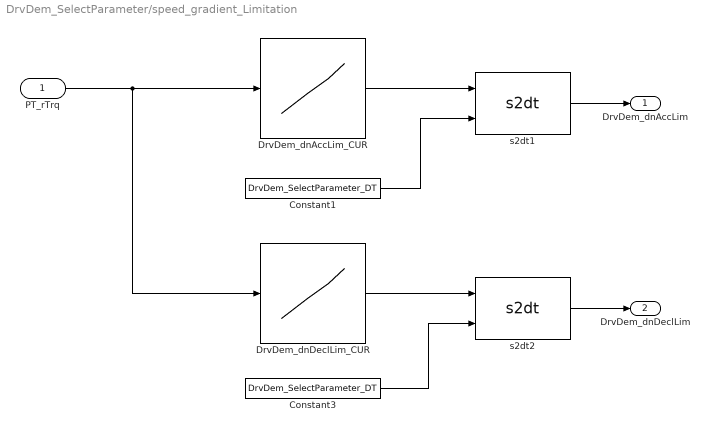
== system DrvDem_SelectParameter/speed_gradient_Limitation ==
  PT_rTrq : Inport
  Constant1 : Constant  Value=DrvDem_SelectParameter_DT  OutDataTypeStr=Inherit: Inherit via back propagation  SampleTime=-1
  Constant3 : Constant  Value=DrvDem_SelectParameter_DT  OutDataTypeStr=Inherit: Inherit via back propagation  SampleTime=-1
  DrvDem_dnAccLim_CUR : Lookup_n-D  NumberOfTableDimensions=1  BreakpointsForDimension1=DrvDem_dnAccLim_CURX  BreakpointsForDimension2=HLSDem_KpCorFac_MAPX  Table=DrvDem_dnAccLim_CUR  ExtrapMethod=Clip  InternalRulePriority=Speed  OutDataTypeStr=Inherit: Inherit via back propagation  RndMeth=Simplest  SaturateOnIntegerOverflow=on
  DrvDem_dnDeclLim_CUR : Lookup_n-D  NumberOfTableDimensions=1  BreakpointsForDimension1=DrvDem_dnDeclLim_CURX  BreakpointsForDimension2=HLSDem_KpCorFac_MAPX  Table=DrvDem_dnDeclLim_CUR  ExtrapMethod=Clip  InternalRulePriority=Speed  OutDataTypeStr=Inherit: Inherit via back propagation  RndMeth=Simplest  SaturateOnIntegerOverflow=on
  s2dt1 : CXLib/s2dt
  s2dt2 : CXLib/s2dt
  DrvDem_dnAccLim : Outport  Tag=rpm/s  Description=Maximum permissible acceleration (Engine speed)  OutMin=-12000  OutMax=12000  OutDataTypeStr=EngSpeed_rpm_s
  DrvDem_dnDeclLim : Outport  Tag=rpm/s  Description=Maximum permissible deceleration (Engine speed)  Port=2  OutMin=-12000  OutMax=12000  OutDataTypeStr=EngSpeed_rpm_s
  wires:
  PT_rTrq/1 -> DrvDem_dnDeclLim_CUR/1, DrvDem_dnAccLim_CUR/1
  s2dt1/1 -> DrvDem_dnAccLim/1
  DrvDem_dnAccLim_CUR/1 -> s2dt1/1
  DrvDem_dnDeclLim_CUR/1 -> s2dt2/1
  s2dt2/1 -> DrvDem_dnDeclLim/1
  Constant3/1 -> s2dt2/2
  Constant1/1 -> s2dt1/2

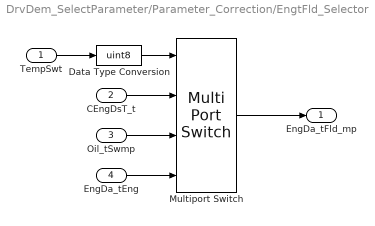
== system DrvDem_SelectParameter/Parameter_Correction/EngtFld_Selector ==
  TempSwt : Inport
  CEngDsT_t : Inport  Tag=deg  Description=engine coolant temperature after filter  Port=2
  Oil_tSwmp : Inport  Tag=deg  Description=Oil temperature in oil sump  Port=3
  EngDa_tEng : Inport  Tag=deg  Description=Engine temperature  Port=4
  Data Type Conversion : DataTypeConversion  OutDataTypeStr=uint8
  Multiport Switch : MultiPortSwitch  DataPortOrder=Zero-based contiguous
  EngDa_tFld_mp : Outport  Tag=deg  Description=Engine temperature field
  wires:
  CEngDsT_t/1 -> Multiport Switch/2
  Multiport Switch/1 -> EngDa_tFld_mp/1
  EngDa_tEng/1 -> Multiport Switch/4
  Oil_tSwmp/1 -> Multiport Switch/3
  Data Type Conversion/1 -> Multiport Switch/1
  TempSwt/1 -> Data Type Conversion/1
